simulink model "untitled"  (R2022b)
settings: Solver=VariableStepAuto  StartTime=0.0  StopTime=10.0  RelTol=1e-3
settings Model: Creator=97083  LastModifiedBy=97083

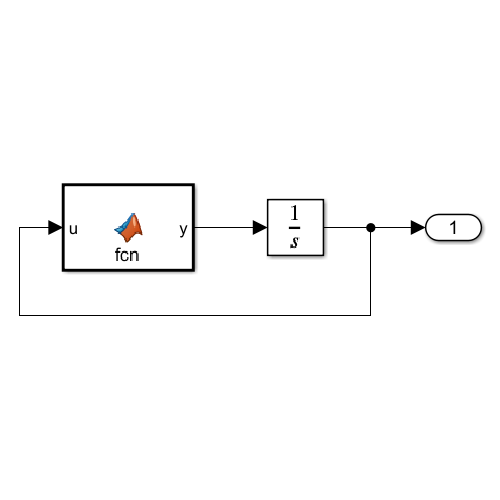
[thumbnail: Simulink's stored preview of the top-level diagram]
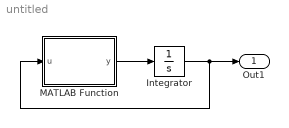
== system untitled ==
  Integrator : Integrator  InitialCondition=[0;0;0];
  MATLAB Function : MATLAB Function  TreatAsAtomicUnit=on
  Out1 : Outport
  wires:
  MATLAB Function/1(y) -> Integrator/1
  Integrator/1 -> MATLAB Function/1(u), Out1/1

== matlab function untitled/MATLAB Function ==
  data: u input; y output
function y = fcn(u)
y=u;
a=0.2;
b=0.2;
c=5.7;
y(1)=-u(2)-u(3);
y(2)=u(1)+a*u(2);
y(3)=b+(u(1)-c)*u(3);
